simulink model "sIMTEO"  (R2025a)
settings: Solver=VariableStepAuto  StartTime=0.0  StopTime=10.0  RelTol=1e-3

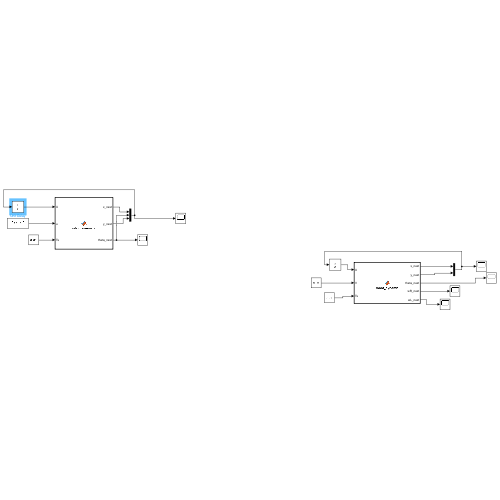
[thumbnail: Simulink's stored preview of the top-level diagram]
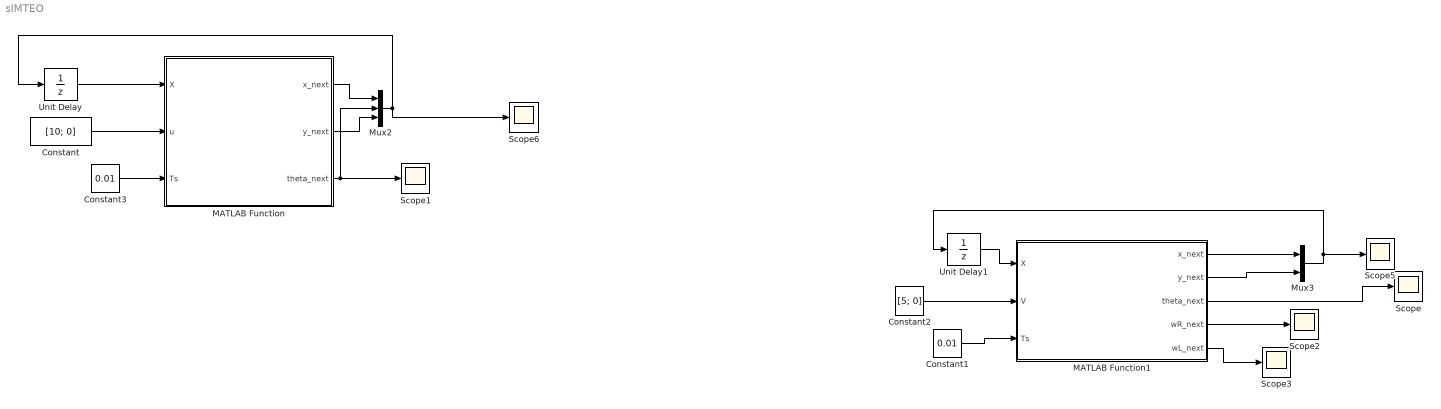
== system sIMTEO ==
  Constant : Constant  Value=[10; 0]
  Constant1 : Constant  Value=0.01
  Constant2 : Constant  Value=[5; 0]
  Constant3 : Constant  Value=0.01
  MATLAB Function : MATLAB Function  TreatAsAtomicUnit=on
  MATLAB Function1 : MATLAB Function  TreatAsAtomicUnit=on
  Mux2 : Mux  Inputs=3
  Mux3 : Mux  Inputs=2
  Scope{,1..3,5..6} (6 alike) : Scope
  Unit Delay : UnitDelay  InitialCondition=[0; 0; 0]  SampleTime=0.01  HasFrameUpgradeWarning=on
  Unit Delay1 : UnitDelay  InitialCondition=[0; 0; 0; 0; 0]  SampleTime=0.01  HasFrameUpgradeWarning=on
  wires:
  Constant/1 -> MATLAB Function/2(u)
  Constant1/1 -> MATLAB Function1/3(Ts)
  Constant2/1 -> MATLAB Function1/2(V)
  Constant3/1 -> MATLAB Function/3(Ts)
  MATLAB Function1/2(y_next) -> Mux3/2
  MATLAB Function1/4(wR_next) -> Scope2/1
  MATLAB Function1/5(wL_next) -> Scope3/1
  MATLAB Function1/3(theta_next) -> Scope/1
  Unit Delay/1 -> MATLAB Function/1(X)
  Unit Delay1/1 -> MATLAB Function1/1(X)
  MATLAB Function/1(x_next) -> Mux2/1
  MATLAB Function/2(y_next) -> Mux2/3
  Mux2/1 -> Scope6/1, Unit Delay/1
  Mux3/1 -> Scope5/1, Unit Delay1/1
  MATLAB Function1/1(x_next) -> Mux3/1
  MATLAB Function/3(theta_next) -> Scope1/1, Mux2/2

== matlab function sIMTEO/MATLAB Function1 ==
function [x_next, y_next, theta_next, wR_next, wL_next] = robot_dynamic(X, V, Ts)
% X = [x; y; theta; wR; wL]
% V = [VR; VL] (V)
% Ts = sample time (s)
% NOTA: copiar/pegar tal cual en el MATLAB Function block de Simulink.

% Parámetros (ajusta con tus valores medidos si quieres)
Kt = 0.03;              % N*m/A
Ke = 0.03;              % V*s/rad
Rm = 2.0;               % Ohm
M_eta = eye(2)*0.01;    % inercia equivalente (2x2) - ajustar si tienes valores
B_eta = 1e-4 * eye(2);  % fricción viscosa (2x2) - ajustar si tienes valores
a = 0.01;               % m per rad
b = 0.05;               % rad per (rad/s)

% Estados actuales
x     = X(1);
y     = X(2);
theta = X(3);
wR    = X(4);
wL    = X(5);

% Modelo eléctrico -> torque (modelo algebraico sin inductancia)
tauR = (Kt / Rm) * (V(1) - Ke * wR);
tauL = (Kt / Rm) * (V(2) - Ke * wL);

% Fricción eléctrica equivalente
B_eq = B_eta + (Kt * Ke / Rm) * eye(2);

% Aceleraciones angulares (vector)
alpha = M_eta \ ([tauR; tauL] - B_eq * [wR; wL]);  % 2x1

% Integrar velocidades angulares (Euler)
wR_next = wR + alpha(1) * Ts;
wL_next = wL + alpha(2) * Ts;

% Cinemática del cuerpo (usar velocidades actuales)
v_body     = a * (wR + wL);
omega_body = b * (wR - wL);   % si wR==wL -> omega_body = 0

% Integrar pose (Euler)
x_next     = x + v_body * cos(theta) * Ts;
y_next     = y + v_body * sin(theta) * Ts;
theta_next = theta + omega_body * Ts;
end

== matlab function sIMTEO/MATLAB Function ==
function [x_next, y_next, theta_next] = robot_kinematic(X, u, Ts)
% X = [x; y; theta]
% u = [wR; wL] (rad/s)
% Ts = sample time (s)
% NOTA: copiar/pegar tal cual en el MATLAB Function block de Simulink.

% Parámetros (ajusta si lo deseas)
a = 0.01;   % m per rad
b = 0.05;   % rad per (rad/s)

% Estados actuales
x     = X(1);
y     = X(2);
theta = X(3);

% Entradas (velocidades angulares de rueda)
wR = u(1);
wL = u(2);

% Cinemática (conveniencia: derecha -> theta positivo)
v_body     = a * (wR + wL);
omega_body = b * (wR - wL);   % si wR==wL -> omega_body = 0

% Integración (Euler forward)
x_next     = x + v_body * cos(theta) * Ts;
y_next     = y + v_body * sin(theta) * Ts;
theta_next = theta + omega_body * Ts;
end
